simulink model "hx_NTU_02_sim"  (R2017b)
settings: Solver=VariableStepAuto  StartTime=0.0  StopTime=0  RelTol=1e-3
libraries: thermochemical x5
settings Model: Creator=fferrucc  LastModifiedBy=fferrucc

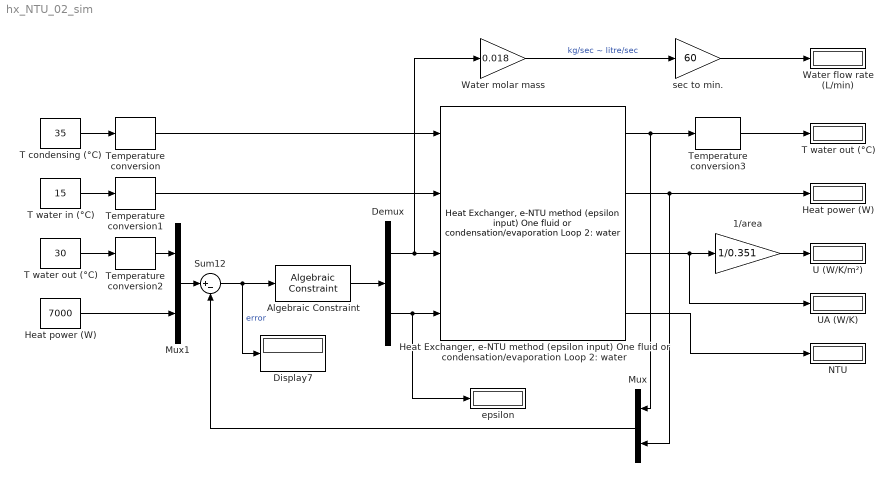
== system hx_NTU_02_sim ==
  1/area : Gain  Gain=1/0.351
  Algebraic Constraint : AlgebraicConstraint  Solver=Trust region  InitialGuess=1
  Demux : Demux  Outputs=2
  Display7 : Display
      settings: Format=short_e
  "Heat Exchanger, e-NTU method (epsilon input) One fluid or condensation/evaporation Loop 2: water" : thermochemical/Heat exchangers/Heat Exchanger, e-NTU method (epsilon input) One fluid or condensation//evaporation Loop 2: water  cp_water_J_K_mol=75.3260
      settings: SourceProductName=@ Thermochemical
  Heat power (W) : Constant  Value=7000
  "Heat power (W) " : Display
  Mux : Mux  Inputs=2
  Mux1 : Mux  Inputs=2
  NTU : Display
  Sum12 : Sum  Inputs=|+-
  T condensing (°C) : Constant  Value=35
  T water in (°C) : Constant  Value=15
  T water out (°C) : Constant  Value=30
  "T water out (°C) " : Display
  Temperature conversion : thermochemical/Conversions/Temperature conversion  sel=°C --> K
      settings: SourceProductName=@ Thermochemical
  Temperature conversion1 : thermochemical/Conversions/Temperature conversion  sel=°C --> K
      settings: SourceProductName=@ Thermochemical
  Temperature conversion2 : thermochemical/Conversions/Temperature conversion  sel=°C --> K
      settings: SourceProductName=@ Thermochemical
  Temperature conversion3 : thermochemical/Conversions/Temperature conversion  sel=K --> °C
      settings: SourceProductName=@ Thermochemical
  U (W/K/m²) : Display
  UA (W/K) : Display
  Water flow rate (L/min) : Display
  Water molar mass : Gain  Gain=0.018
  epsilon : Display
  sec to min. : Gain  Gain=60
  wires:
  "Heat Exchanger, e-NTU method (epsilon input) One fluid or condensation/evaporation Loop 2: water"/1 -> Temperature conversion3/1, Mux/1
  "Heat Exchanger, e-NTU method (epsilon input) One fluid or condensation/evaporation Loop 2: water"/2 -> "Heat power (W) "/1, Mux/2
  "Heat Exchanger, e-NTU method (epsilon input) One fluid or condensation/evaporation Loop 2: water"/4 -> NTU/1
  T condensing (°C)/1 -> Temperature conversion/1
  Temperature conversion/1 -> "Heat Exchanger, e-NTU method (epsilon input) One fluid or condensation/evaporation Loop 2: water"/1
  T water in (°C)/1 -> Temperature conversion1/1
  Temperature conversion1/1 -> "Heat Exchanger, e-NTU method (epsilon input) One fluid or condensation/evaporation Loop 2: water"/2
  T water out (°C)/1 -> Temperature conversion2/1
  Temperature conversion2/1 -> Mux1/1
  Heat power (W)/1 -> Mux1/2
  Temperature conversion3/1 -> "T water out (°C) "/1
  "Heat Exchanger, e-NTU method (epsilon input) One fluid or condensation/evaporation Loop 2: water"/3 -> UA (W/K)/1, 1/area/1
  1/area/1 -> U (W/K/m²)/1
  Mux1/1 -> Sum12/1
  Mux/1 -> Sum12/2
  Sum12/1 -> Display7/1, Algebraic Constraint/1  "error"
  Algebraic Constraint/1 -> Demux/1
  Demux/2 -> epsilon/1, "Heat Exchanger, e-NTU method (epsilon input) One fluid or condensation/evaporation Loop 2: water"/4
  Demux/1 -> Water molar mass/1, "Heat Exchanger, e-NTU method (epsilon input) One fluid or condensation/evaporation Loop 2: water"/3
  Water molar mass/1 -> sec to min./1  "kg/sec ~ litre/sec"
  sec to min./1 -> Water flow rate (L/min)/1
